simulink model "result2"  (R2020a)
settings: Solver=VariableStepAuto  StartTime=0.0  StopTime=10.0  RelTol=1e-3
settings Model: Creator=ASUS  LastModifiedBy=ASUS

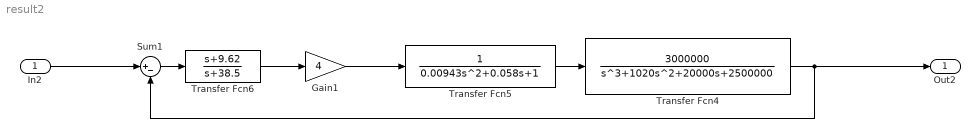
== system result2 ==
  In2 : Inport
  Gain1 : Gain  Gain=4
  Sum1 : Sum  Inputs=|+-
  Transfer Fcn4 : TransferFcn  Numerator=[3000000]  Denominator=[1 1020 20000 2500000]
  Transfer Fcn5 : TransferFcn  Denominator=[0.00943 0.058 1]
  Transfer Fcn6 : TransferFcn  Numerator=[1 9.62]  Denominator=[1 38.5]
  Out2 : Outport
  wires:
  Transfer Fcn5/1 -> Transfer Fcn4/1
  Transfer Fcn6/1 -> Gain1/1
  Gain1/1 -> Transfer Fcn5/1
  In2/1 -> Sum1/1
  Transfer Fcn4/1 -> Out2/1, Sum1/2
  Sum1/1 -> Transfer Fcn6/1
